simulink model "TST_SfFunctionWithBusTypes"  (Simulink 7.4)
settings: Solver=FixedStepDiscrete  StartTime=0.0  StopTime=10.0  FixedStep=0.02  RelTol=1e-3
settings Model: Creator=kharthforeign  LastModifiedBy=kharthforeign  BufferReuse=off
settings DataIOCC: SaveOutput=off  SignalLogging=off  SaveTime=off
settings OptimizationCC: BlockReduction=off  ConditionallyExecuteInputs=off  OptimizeBlockIOStorage=off  BufferReuse=off  ExpressionFolding=off  LocalBlockOutputs=off  InitFltsAndDblsToZero=on

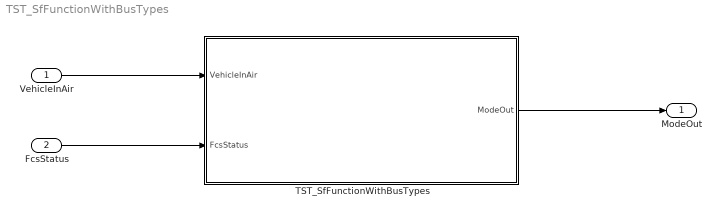
== system TST_SfFunctionWithBusTypes ==
  VehicleInAir : Inport  PortDimensions=1  DataType=boolean  OutDataType=fixdt(1, 16)  OutScaling=2^0  OutDataTypeStr=boolean
  FcsStatus : Inport  Port=2  UseBusObject=on  OutDataType=fixdt(1, 16)  OutScaling=2^0
      settings: BusObject=FCS_FlightControlSystem_Status
  TST_SfFunctionWithBusTypes : Subsystem  TreatAsAtomicUnit=on
  ModeOut : Outport  PortDimensions=1  DataType=uint32  OutDataType=Enum: GBL_Definitions_EjectionCmd  OutDataTypeStr=uint32
  wires:
  VehicleInAir/1 -> TST_SfFunctionWithBusTypes/1(VehicleInAir)
  FcsStatus/1 -> TST_SfFunctionWithBusTypes/2(FcsStatus)
  TST_SfFunctionWithBusTypes/1(ModeOut) -> ModeOut/1

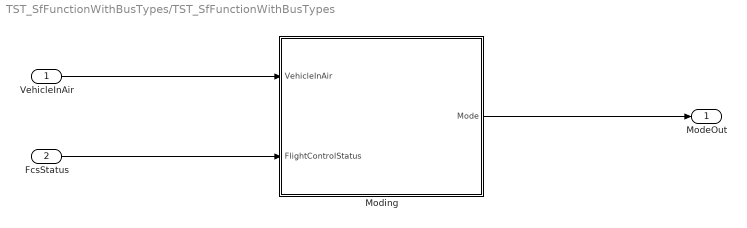
== system TST_SfFunctionWithBusTypes/TST_SfFunctionWithBusTypes ==
  VehicleInAir : Inport  PortDimensions=1  DataType=boolean  OutDataType=fixdt(1, 16)  OutScaling=2^0  OutDataTypeStr=boolean
  FcsStatus : Inport  Port=2  UseBusObject=on  OutDataType=fixdt(1, 16)  OutScaling=2^0
      settings: BusObject=FCS_FlightControlSystem_Status
  Moding : Stateflow chart  TreatAsAtomicUnit=on
  ModeOut : Outport  PortDimensions=1  DataType=uint32  OutDataType=Enum: GBL_Definitions_EjectionCmd  OutDataTypeStr=uint32
  wires:
  FcsStatus/1 -> Moding/2(FlightControlStatus)
  VehicleInAir/1 -> Moding/1(VehicleInAir)
  Moding/1(Mode) -> ModeOut/1

== stateflow chart TST_SfFunctionWithBusTypes/Moding ==
  state UpdateFeedthroughParameters(FcsStatusInput) [function]
    (default) -> (junction 5)
    (junction 5) -> (junction 6) [order 2] : {Mode = uint32(5);}
    (junction 5) -> (junction 7) [order 1] : [FcsStatusInput.PressureAltitude_Ft > 5000.0]...
        | {Mode = uint32(5);}
  state Main
    entry:
    UpdateFeedthroughParameters(FlightControlStatus);
  (default) -> Main
  data: FcsStatusInput function_input FCS_FlightControlSystem_Status; VehicleInAir input boolean; Mode output uint32; FlightControlStatus input FCS_FlightControlSystem_Status
